simulink model "Chap8_2sim"  (R2019a)
settings: Solver=VariableStepAuto  StartTime=0.0  StopTime=20  MaxStep=.01  RelTol=1e-3
settings Model: Creator=zkibria  LastModifiedBy=zkibria

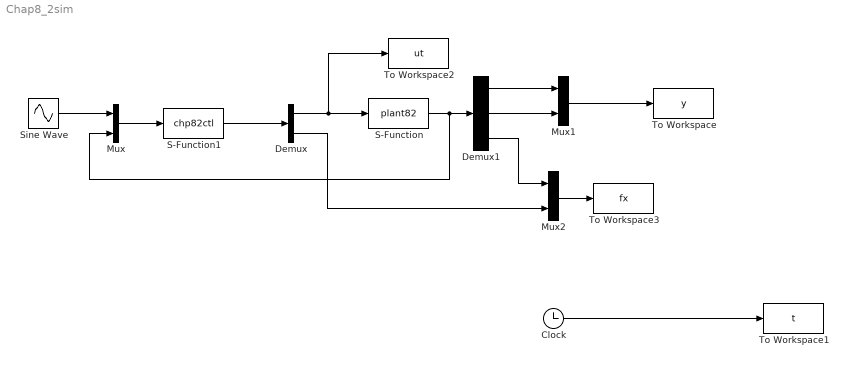
== system Chap8_2sim ==
  Clock : Clock
  Demux : Demux  Outputs=2
  Demux1 : Demux  Outputs=3
  Mux : Mux  Inputs=2
  Mux1 : Mux  Inputs=2
  Mux2 : Mux  Inputs=2
  S-Function : S-Function  FunctionName=plant82  SFunctionDeploymentMode=off  EnableBusSupport=off
  S-Function1 : S-Function  FunctionName=chp82ctl  SFunctionDeploymentMode=off  EnableBusSupport=off
  Sine Wave : Sin  SampleTime=0
  To Workspace : ToWorkspace  VariableName=y  SaveFormat=Timeseries  SampleTime=-1
  To Workspace1 : ToWorkspace  VariableName=t  SaveFormat=Timeseries  SampleTime=-1
  To Workspace2 : ToWorkspace  VariableName=ut  SaveFormat=Timeseries  SampleTime=-1
  To Workspace3 : ToWorkspace  VariableName=fx  SaveFormat=Timeseries  SampleTime=-1
  wires:
  Clock/1 -> To Workspace1/1
  Sine Wave/1 -> Mux/1
  Mux/1 -> S-Function1/1
  S-Function1/1 -> Demux/1
  Demux/1 -> To Workspace2/1, S-Function/1
  S-Function/1 -> Mux/2, Demux1/1
  Demux1/1 -> Mux1/1
  Demux1/2 -> Mux1/2
  Mux1/1 -> To Workspace/1
  Demux1/3 -> Mux2/1
  Demux/2 -> Mux2/2
  Mux2/1 -> To Workspace3/1
